simulink model "Mass_Springs_Systems"  (R2021b)
settings: Solver=daessc  StartTime=0.0  StopTime=20  FixedStep=.001  RelTol=1e-3  AbsTol=1e-3  EnableMultiTasking=on
model workspace (MAT data in the model file):
  cslide = 0.25
  iz = [0.192 0.207 0.221 0.238 0.251 0.262 0.268 0.27 0.267 0.262 0.246 0.232 ... (50 elements, 25x2)]
  m1 = 0
  m2 = 0
  m3 = 0
  one = [0.064  0.072; 0.088  0.03; 0.169  0.03; 0.168  0.458; 0.129  0.458; 0.128  0.073]
  smiData : object (value not decoded)
  three = [0.252 0.239 0.214 0.179 0.14 0.107 0.083 0.065 0.075 0.102 0.129 0.163 ... (112 elements, 56x2)]
  two = [0.081 0.042 0.05 0.06 0.082 0.106 0.135 0.161 0.194 0.226 0.253 0.279 ... (72 elements, 36x2)]
  xy_simple = [39.1661  19.7032018238; 3.8339  19.7032; -0.28263658  19.7032; -0.28263658  0; 43  0; 43  19.7032]
  zero = [0.2 0.245 0.288 0.316 0.335 0.345 0.347 0.344 0.338 0.324 0.3 0.269 ... (50 elements, 25x2)]
undefined symbols (not defined in the file): A, d1, d2, ha, sigbuilder_block, X, Y, Z
libraries: sm_lib x7213, nesl_utility x58, simulink x1
(part 2 of 146)

== system Mass_Springs_Systems/Mass Spring Damper Systems ==
  note: 1 Mass 1 Spring
  note: 3 Mass 3 Spring
  note: 2 Mass 2 Spring
  note: 1 Mass 2 Spring
  note: 2 Mass 3 Spring
  note: Equivalent System
  note: Vibrational Machine
  2Masses 2Springs : Subsystem  AncestorBlock=Lib/2Masses 2Springs  VariantControl=22ms  mask{m1=2, m2=1, k1=600, k2=400, d=1, s_f=.35, id1=2, id2=2, zero_forces=on, zerodis=off, force_type=Harmonic, Force=1, Har_Force=1, freq=sqrt(400/1.5)}
      mask prompts: m1 "Mass1 (kg)"; m2 "Mass2 (kg)"; k1 "K1 Spring Constant (N/m)"; k2 "K2 Spring Constant (N/m)"; d "Spring Damping (kg/s)"; s_f "Surface Friction (N/(m/s))"; id1 "M1 Initial Displacement (cm)"; id2 "M2 Initial Displacement (cm)"; zero_forces "Zero Forces"; zerodis "Zero Initial Displacement"; force_type "Force Response Type"; Force "Magnitude(N)"; Har_Force "Magnitude(N)"; freq "Frequency(rad/s)"
      mask init:
      | switch force_type
      |     case 1
      |         Har_Force = 0;
      |         freq = 0;
      |     case 2
      |         Force = 0;
      | end
      | if zero_forces == 1
      |     Har_Force = 0;
      |     Force = 0;
      |     freq = 0;
      | end
      | 
      | if zerodis == 1
      |     id1=0;
      |     id2=0;
      | end
      mask Callback zero_forces:
      | % Enable and disable parameters
      | 
      | % Get the value of the Enable Bias checkbox
      | % unchecked = 'off'
      | % checked = 'on'
      | enab = get_param(gcb,'zero_forces');
      | 
      | % Set the 'MaskEnables' property for each parameters
      | if strcmp(enab,'on')
      |     set_param(gcb,'MaskVisibilities',{'on','on','on','on','on','on','on','on','on','off','off','off','off','off'});
      | else
      |     set_param(gcb,'MaskVisibilities',{'on','on','on','on','on','on','on','on','on','on','on','on','on','on'});
      | end
      | 
      | % Note that the value of the bias is not handled here.
      | % See the Initialization tab
      mask Callback zerodis:
      | % Enable and disable parameters
      | 
      | % Get the value of the Enable Bias checkbox
      | % unchecked = 'off'
      | % checked = 'on'
      | enab = get_param(gcb,'zerodis');
      | 
      | % Set the 'MaskEnables' property for each parameters
      | if strcmp(enab,'on')
      |     set_param(gcb,'MaskEnables',{'on','on','on','on','on','on','off','off','on','on','on','on','on','on'});
      | else
      |     set_param(gcb,'MaskEnables',{'on','on','on','on','on','on','on','on','on','on','on','on','on','on'});
      | end
      | 
      | % Note that the value of the bias is not handled here.
      | % See the Initialization tab
      mask TypeOptions force_type: Step | Harmonic
      mask DialogControl Control4 Prompt: Update Model
      mask DialogControl Control4 Callback: set_param(bdroot,'SimulationCommand','update')
      mask DialogControl Control2 Prompt: Run Simulation
      mask DialogControl Control2 Callback: set_param(bdroot,'SimulationCommand','start')
      mask DialogControl Control3 Prompt: STOP Simulation
      mask DialogControl Control3 Callback: set_param(bdroot,'SimulationCommand','stop')
      mask DialogControl Control7 Prompt: Open Scope Plot
      mask DialogControl Control7 Callback: open(Simulink.BlockPath({'Mass_Springs_Systems/Mass Spring Damper Systems/2Masses 2Springs/Position'}))
      mask DialogControl Control14 Prompt: Frequency Plot
      mask DialogControl Control14 Callback:
      | cart1=evalin('base','out.pos1');
      | cart2=evalin('base','out.pos2');
      | time=evalin('base','out.tout');
      | 
      | Ts = time(2)-time(1);
      | fs = 1/Ts;
      | N = length(cart1);
      | 
      | Y1 = abs(fft(cart1)/N); % fft of cart1 data
      | Y1d = Y1(1:N/2+1); %single side spectrum
      | Y1d(2:end-1) = 2*Y1d(2:end-1); %amplitude adjustment
      | 
      | Y2 = abs(fft(cart2)/N);
      | Y2d = Y2(1:N/2+1);
      | Y2d(2:end-1) = 2*Y2d(2:end-1);
      | 
      | 
      | f = fs*(0:(N/2))/N; %create frequency vector
      | 
      | figure;
      | plot(f,Y1d); xlim([0 10]);
      | hold on;
      | plot(f,Y2d,'r')
      | hold off;
      mask DialogControl Control16 Prompt: Mode Ratios
      mask DialogControl Control16 Callback:
      | syms  w
      | m1=get_param(gcb,'m1');
      | m1=str2double(m1);
      | m2=get_param(gcb,'m2');
      | m2=str2double(m2);
      | k1=get_param(gcb,'k1');
      | k1=str2double(k1);
      | k2=get_param(gcb,'k2');
      | k2=str2double(k2);
      | M=[k1+k2-m1*w^2 -k2; -k2 k2-m2*w^2];
      | detM=det(M);
      | solution=double(solve(detM==0,w));
      | pos=solution>0;
      | wsolution=solution(pos);
      | w1=wsolution(1);
      | w2=wsolution(2);
      | f1=w1/(2*pi);
      | f2=w2/(2*pi);
      | M1=double(subs(M,w,w1));
      | Mode_Ratio_1=M1(1,1)/-M1(1,2);
      | M2=double(subs(M,w,w2));
      | Mode_Ratio_2=M2(1,1)/-M2(1,2);
      | %set_param(gcb,'MaskSelfModifiable','on');
      | % Get the mask object
      | mo = get_param(gcb,'MaskObject');
      | % Get the text object
      | tc = mo.getDialogControl('TextControl1');
      | % Change the string
      | tc.Prompt = string(Mode_Ratio_1);
      | % Get the text object
      | tc = mo.getDialogControl('TextControl2');
      | % Change the string
      | tc.Prompt = string(Mode_Ratio_2);
      mask DialogControl Container6 Prompt: Variables
      mask DialogControl Control13 Prompt: (Add text here)
      mask DialogControl Container8 Prompt: Free Response
      mask DialogControl Container11 Prompt: Free Response
      mask DialogControl Control17 Prompt: Mode Ratio of Mass 1:
      mask DialogControl TextControl1 Prompt: 1.6861
      mask DialogControl Control19 Prompt: Mode Ratio of Mass 2:
      mask DialogControl TextControl2 Prompt: -1.1861
      mask DialogControl Control10 Prompt: "Check Box below for Only Free Response"
      mask DialogControl Container19 Prompt: Forced Response
      mask DialogControl Container10 Prompt: Forced Response
      mask DialogControl Control9 Prompt: Uncheck "Zero Forces" in Free Response Tab to add Forced Response
      mask DialogControl Container13 Prompt: Step Response
      mask DialogControl Container16 Prompt: Harmonic Response
      mask Display: image('$imagefile'); % Use "Edit Image" on toolstrip to change.
  2Masses 3Springs : Subsystem  AncestorBlock=Lib/2Masses 3Springs  VariantControl=23ms  mask{m1=2, m2=2, k1=700, k2=300, k3=700, d=1/3, s_f=0, id1=3.500, id2=-3.500, zero_forces=on, zerodis=off, force_type=Harmonic, Force=5, Har_Force=3, freq=20}
      mask prompts: m1 "Mass1 (kg)"; m2 "Mass2 (kg)"; k1 "K1 Spring Constant (N/m)"; k2 "K2 Spring Constant (N/m)"; k3 "K3 Spring Constant (N/m)"; d "Spring Damping (kg/s)"; s_f "Surface Friction (N/(m/s))"; id1 "M1 Initial Displacement (cm)"; id2 "M2 Initial Displacement (cm)"; zero_forces "Zero Forces"; zerodis "Zero Initial Displacement"; force_type "Force Response Type"; Force "Magnitude(N)"; Har_Force "Magnitude(N)"; freq "Frequency(rad/s)"
      mask init:
      | switch force_type
      |     case 1
      |         Har_Force = 0;
      |         freq = 0;
      |     case 2
      |         Force = 0;
      | end
      | if zero_forces == 1
      |     Har_Force = 0;
      |     Force = 0;
      |     freq = 0;
      | end
      | 
      | if zerodis == 1
      |     id1 = 0;
      |     id2 = 0;
      | end
      mask Callback zero_forces:
      | % Enable and disable parameters
      | 
      | % Get the value of the Enable Bias checkbox
      | % unchecked = 'off'
      | % checked = 'on'
      | enab = get_param(gcb,'zero_forces');
      | 
      | % Set the 'MaskEnables' property for each parameters
      | if strcmp(enab,'on')
      |     set_param(gcb,'MaskVisibilities',{'on','on','on','on','on','on','on','on','on','on','off','off','off','off','off'});
      | else
      |     set_param(gcb,'MaskVisibilities',{'on','on','on','on','on','on','on','on','on','on','on','on','on','on','on'});
      | end
      | 
      | % Note that the value of the bias is not handled here.
      | % See the Initialization tab
      mask Callback zerodis:
      | % Enable and disable parameters
      | 
      | % Get the value of the Enable Bias checkbox
      | % unchecked = 'off'
      | % checked = 'on'
      | enab = get_param(gcb,'zerodis');
      | 
      | % Set the 'MaskEnables' property for each parameters
      | if strcmp(enab,'on')
      |     set_param(gcb,'MaskEnables',{'on','on','on','on','on','on','on','off','off','on','on','on','on','on','on'});
      | else
      |     set_param(gcb,'MaskEnables',{'on','on','on','on','on','on','on','on','on','on','on','on','on','on','on'});
      | end
      | 
      | % Note that the value of the bias is not handled here.
      | % See the Initialization tab
      mask TypeOptions force_type: Step | Harmonic
      mask DialogControl Control4 Prompt: Update Model
      mask DialogControl Control4 Callback: set_param(bdroot,'SimulationCommand','update')
      mask DialogControl Control14 Prompt: Run Simulation
      mask DialogControl Control14 Callback: set_param(bdroot,'SimulationCommand','start')
      mask DialogControl Control3 Prompt: STOP Simulation
      mask DialogControl Control3 Callback: set_param(bdroot,'SimulationCommand','stop')
      mask DialogControl Control7 Prompt: Open Scope Plot
      mask DialogControl Control7 Callback: open(Simulink.BlockPath({'Mass_Springs_Systems/Mass Spring Damper Systems/2Masses 3Springs/Position'}))
      mask DialogControl Control15 Prompt: Frequency Plot
      mask DialogControl Control15 Callback:
      | cart1=evalin('base','out.pos1');
      | cart2=evalin('base','out.pos2');
      | time=evalin('base','out.tout');
      | 
      | Ts = time(2)-time(1);
      | fs = 1/Ts;
      | N = length(cart1);
      | 
      | Y1 = abs(fft(cart1)/N); % fft of cart1 data
      | Y1d = Y1(1:N/2+1); %single side spectrum
      | Y1d(2:end-1) = 2*Y1d(2:end-1); %amplitude adjustment
      | 
      | Y2 = abs(fft(cart2)/N);
      | Y2d = Y2(1:N/2+1);
      | Y2d(2:end-1) = 2*Y2d(2:end-1);
      | 
      | 
      | f = fs*(0:(N/2))/N; %create frequency vector
      | 
      | figure;
      | plot(f,Y1d); xlim([0 10]);
      | hold on;
      | plot(f,Y2d,'r')
      mask DialogControl Control18 Prompt: Mode Ratios
      mask DialogControl Control18 Callback:
      | syms  w
      | m1=get_param(gcb,'m1');
      | m1=str2double(m1);
      | m2=get_param(gcb,'m2');
      | m2=str2double(m2);
      | k1=get_param(gcb,'k1');
      | k1=str2double(k1);
      | k2=get_param(gcb,'k2');
      | k2=str2double(k2);
      | k3=get_param(gcb,'k3');
      | k3=str2double(k3);
      | M=[k1+k2-m1*w^2 -k2; -k2 k2+k3-m2*w^2];
      | detM=det(M);
      | solution=double(solve(detM==0,w));
      | pos=solution>0;
      | wsolution=solution(pos);
      | w1=wsolution(1);
      | w2=wsolution(2);
      | f1=w1/(2*pi);
      | f2=w2/(2*pi);
      | M1=double(subs(M,w,w1)) ;
      | Mode_Ratio_1=M1(1,1)/-M1(1,2);
      | M2=double(subs(M,w,w2)) ;
      | Mode_Ratio_2=M2(1,1)/-M2(1,2);
      | %set_param(gcb,'MaskSelfModifiable','on');
      | % Get the mask object
      | mo = get_param(gcb,'MaskObject');
      | % Get the text object
      | tc = mo.getDialogControl('TextControl1');
      | % Change the string
      | tc.Prompt = string(Mode_Ratio_1);
      | % Get the text object
      | tc = mo.getDialogControl('TextControl2');
      | % Change the string
      | tc.Prompt = string(Mode_Ratio_2);
      mask DialogControl Container6 Prompt: Variables
      mask DialogControl Container8 Prompt: Free Response
      mask DialogControl Container11 Prompt: Free Response
      mask DialogControl Control21 Prompt: Mode Ratio of Mass1:
      mask DialogControl TextControl1 Prompt: 1
      mask DialogControl Control22 Prompt: Mode Ratio of Mass 2:
      mask DialogControl TextControl2 Prompt: -1
      mask DialogControl Control10 Prompt: "Check Box below for Only Free Response"
      mask DialogControl Container19 Prompt: Forced Response
      mask DialogControl Container10 Prompt: Forced Response
      mask DialogControl Control9 Prompt: Uncheck "Zero Forces" in Free Response Tab to add Forced Response
      mask DialogControl Container13 Prompt: Step Response
      mask DialogControl Container16 Prompt: Harmonic Response
      mask Display: image('$imagefile'); % Use "Edit Image" on toolstrip to change.
  3Masses 3Springs : Subsystem  AncestorBlock=Lib/3Masses 3Springs  VariantControl=33ms  mask{m1=1, m2=1, m3=1, k1=100, k2=100, k3=100, d=1, s_f=0, d1=3.500, d2=3.500, d3=3.500, zero_forces=off, zerodis=off, force_type=Step, Force=5, Har_Force=6, freq=20}
      mask prompts: m1 "Mass1 (kg)"; m2 "Mass2 (kg)"; m3 "Mass3 (kg)"; k1 "K1 Spring Constant (N/m)"; k2 "K2 Spring Constant (N/m)"; k3 "K3 Spring Constant (N/m)"; d "Spring Damping (kg/s)"; s_f "Surface Friction (N/(m/s))"; d1 "M1 Initial Displacement (cm)"; d2 "M2 Initial Displacement (cm)"; d3 "M3 Initial Displacement (cm)"; zero_forces "Zero Forces"; zerodis "Zero Initial Displacement"; force_type "Force Response Type"; Force "Magnitude(N)"; Har_Force "Magnitude(N)"; freq "Frequency(rad/s)"
      mask init:
      | switch force_type
      |     case 1
      |         Har_Force = 0;
      |         freq = 0;
      |     case 2
      |         Force = 0;
      | end
      | if zero_forces == 1
      |     Har_Force = 0;
      |     Force = 0;
      |     freq = 0;
      | end
      | 
      | if zerodis == 1
      |     id1 = 0;
      |     id2 = 0;
      |     id3 = 0;
      | end
      mask Callback zero_forces:
      | % Enable and disable parameters
      | 
      | % Get the value of the Enable Bias checkbox
      | % unchecked = 'off'
      | % checked = 'on'
      | enab = get_param(gcb,'zero_forces');
      | 
      | % Set the 'MaskEnables' property for each parameters
      | if strcmp(enab,'on')
      |     set_param(gcb,'MaskVisibilities',{'on','on','on','on','on','on','on','on','on','on','on','on','off','off','off','off','off'});
      | else
      |     set_param(gcb,'MaskVisibilities',{'on','on','on','on','on','on','on','on','on','on','on','on','on','on','on','on','on'});
      | end
      | 
      | % Note that the value of the bias is not handled here.
      | % See the Initialization tab
      mask Callback zerodis:
      | % Enable and disable parameters
      | 
      | % Get the value of the Enable Bias checkbox
      | % unchecked = 'off'
      | % checked = 'on'
      | enab = get_param(gcb,'zerodis');
      | 
      | % Set the 'MaskEnables' property for each parameters
      | if strcmp(enab,'on')
      |     set_param(gcb,'MaskEnables',{'on','on','on','on','on','on','on','on','off','off','off','on','on','on','on','on','on'});
      | else
      |     set_param(gcb,'MaskEnables',{'on','on','on','on','on','on','on','on','on','on','on','on','on','on','on','on','on'});
      | end
      | 
      | % Note that the value of the bias is not handled here.
      | % See the Initialization tab
      mask TypeOptions force_type: Step | Harmonic
      mask DialogControl Control4 Prompt: Update Model
      mask DialogControl Control4 Callback: set_param(bdroot,'SimulationCommand','update')
      mask DialogControl Control2 Prompt: Run Simulation
      mask DialogControl Control2 Callback: set_param(bdroot,'SimulationCommand','start')
      mask DialogControl Control3 Prompt: STOP Simulation
      mask DialogControl Control3 Callback: set_param(bdroot,'SimulationCommand','stop')
      mask DialogControl Control7 Prompt: Open Scope Plot
      mask DialogControl Control7 Callback: open(Simulink.BlockPath({'Mass_Springs_Systems/Mass Spring Damper Systems/3Masses 3Springs/Position'}))
      mask DialogControl Control14 Prompt: Frequency Plot
      mask DialogControl Control14 Callback:
      | cart1=evalin('base','out.pos1');
      | cart2=evalin('base','out.pos2');
      | cart3=evalin('base','out.pos3');
      | time=evalin('base','out.tout');
      | 
      | Ts = time(2)-time(1);
      | fs = 1/Ts;
      | N = length(cart1);
      | 
      | Y1 = abs(fft(cart1)/N); % fft of cart1 data
      | Y1d = Y1(1:N/2+1); %single side spectrum
      | Y1d(2:end-1) = 2*Y1d(2:end-1); %amplitude adjustment
      | 
      | Y2 = abs(fft(cart2)/N);
      | Y2d = Y2(1:N/2+1);
      | Y2d(2:end-1) = 2*Y2d(2:end-1);
      | 
      | Y3 = abs(fft(cart3)/N);
      | Y3d = Y3(1:N/2+1);
      | Y3d(2:end-1) = 2*Y3d(2:end-1);
      | 
      | f = fs*(0:(N/2))/N; %create frequency vector
      | 
      | figure;
      | plot(f,Y1d); xlim([0 10]);
      | hold on;
      | plot(f,Y2d,'r')
      | plot(f,Y3d,'g')
      mask DialogControl Container6 Prompt: Variables
      mask DialogControl Container8 Prompt: Free Response
      mask DialogControl Container11 Prompt: Free Response
      mask DialogControl Control10 Prompt: "Check Box below for Only Free Response"
      mask DialogControl Container19 Prompt: Forced Response
      mask DialogControl Container10 Prompt: Forced Response
      mask DialogControl Control9 Prompt: Uncheck "Zero Forces" in Free Response Tab to add Forced Response
      mask DialogControl Container13 Prompt: Step Response
      mask DialogControl Container16 Prompt: Harmonic Response
      mask Display: image('$imagefile'); % Use "Edit Image" on toolstrip to change.
  Equivalent System : Subsystem  VariantControl=ES  mask{length=20, b_thk=2.8, tip_mass=0, materials=TPU, den=.88, ymod=3.5, pr=.3, t_spr1=off, top_spr1_stiff=10, top_spr1_dpg=0, t_spr2=off, top_spr2_stiff=50, top_spr2_dpg=.00001, t_spr3=off, top_spr3_stiff=20, top_spr3_dpg=0, t_spr4=on, top_spr4_stiff=50, top_spr4_dpg=.00001, b_spr1=off, bottom_spr1_stiff=10, bottom_spr1_dpg=1, b_spr2=off, bottom_spr2_stiff=0, bottom_spr2_dpg=0, b_spr3=off, bottom_spr3_stiff=.5, bottom_spr3_dpg=0.00001, b_spr4=off, bottom_spr4_stiff=.5, bottom_spr4_dpg=0, theta=-4.800, zerodis=off, freeforce=on, type_force=Harmonic, Force=2, Har_Force=2, freq=5, Imp_Force=1, meq=1, keq=100, ceq=1}
      mask prompts: length "Beam Length (cm)"; b_thk "Beam Thickness (mm)"; tip_mass "Load Mass (g)"; materials "Beam Material"; den "Density (g/cm^3)"; ymod "Young's Modulus (GPa)"; pr "Poisson's Ratio"; t_spr1 "Spring 1"; top_spr1_stiff "Stiffness (N/m)"; top_spr1_dpg "Damping (N/m)"; t_spr2 "Spring 2"; top_spr2_stiff "Stiffness (N/m)"; top_spr2_dpg "Damping (N/m)"; t_spr3 "Spring 3"; top_spr3_stiff "Stiffness (N/m)"; top_spr3_dpg "Damping (N/m)"; t_spr4 "Spring 4"; top_spr4_stiff "Stiffness (N/m)"; top_spr4_dpg "Damping (N/m)"; b_spr1 "Spring 1"; bottom_spr1_stiff "Stiffness (N/m)"; bottom_spr1_dpg "Damping (N/m)"; b_spr2 "Spring 2"; bottom_spr2_stiff "Stiffness (N/m)"; bottom_spr2_dpg "Damping (N/m)"; b_spr3 "Spring 3"; bottom_spr3_stiff "Stiffness (N/m)"; bottom_spr3_dpg "Damping (N/m)"; b_spr4 "Spring 4"; bottom_spr4_stiff "Stiffness (N/m)"; bottom_spr4_dpg "Damping (N/m)"; theta "Inital Displacement of Beam (deg):"; zerodis "Zero Initial Displacement"; freeforce "Zero Forces"; type_force "Force Response Type"; Force "Magnitude (N):"; Har_Force "Magnitude (N):"; freq "Frequency (rad/s):"; Imp_Force "Magnitude (N):"; meq "Equivalent Mass (kg):"; keq "Equivalent Stiffness (N/m):"; ceq "Equivalent Damping (N/m):"
      mask init:
      | t1ih=(1/4)*length*tand(-theta)*.01;
      | t2ih=(2/4)*length*tand(-theta)*.01;
      | t3ih=(3/4)*length*tand(-theta)*.01;
      | t4ih=length*tand(-theta)*.01;
      | b1ih=(1/4)*length*tand(theta)*.01;
      | b2ih=(2/4)*length*tand(theta)*.01;
      | b3ih=(3/4)*length*tand(theta)*.01;
      | b4ih=length*tand(theta)*.01;
      | 
      | thetaeq = -length*tand(theta)*.01;
      | switch materials
      |     case 1
      |         b_stff = 259;
      |         b_damping = .013;
      |         b_density= 7.85;
      | %        b_ymod= 200e9;
      | %         b_pr= .285;
      |     case 2
      |         b_stff = 3.27;
      |         b_damping = .00056;
      |         b_density= 1.2;
      | %        b_ymod= 2.53e9;
      | %         b_pr= .33;
      |     case 3
      |         b_stff = 4.522;
      |         b_damping = .000675;
      |         b_density= 1.24;
      | %        b_ymod= 3.5e9;
      | %         b_pr= .3;
      |     case 4
      |         b_stff = 2.59725;
      |         b_damping = .000515;
      |         b_density= 1.23;
      | %        b_ymod= 2.01e9;
      | %         b_pr= .32;
      |     case 5
      |         Ia = (.025*(b_thk*10^-3)^3)/12;
      |         l = length*10^-2/4;
      |         b_stff = (ymod*10^9*Ia)/l;
      |         b_damping = .0001*2*b_stff;
      |         b_density = den;
      | end
      | switch type_force
      |     case 1,
      |         Imp_Force=0;
      |         Har_Force=0;
      |         freq=0;
      |     case 2,
      |         Force=0;
      |         Imp_Force=0;
      |     case 3
      |         Force=0;
      |         Har_Force=0;
      |         freq=0;
      |     otherwise, assert(false);
      | end
      | if freeforce == 1
      |     Force = 0;
      |     Har_Force = 0;
      |     Imp_Force = 0;
      | end
      | 
      | if zerodis == 1
      |     t1ih= 0;
      |     t2ih= 0;
      |     t3ih= 0;
      |     t4ih= 0;
      |     b1ih= 0;
      |     b2ih= 0;
      |     b3ih= 0;
      |     b4ih= 0;
      |     theta=0;
      | end
      mask TypeOptions materials: Steel | TPU | PLA | PETG | Enter Material Properties
      mask Callback materials:
      | %Getting cell of blocks
      | parnum1 = find(strcmp(get_param('Mass_Springs_Systems/Mass Spring Damper Systems/Equivalent System','MaskNames'),'den'));
      | parnum2 = find(strcmp(get_param('Mass_Springs_Systems/Mass Spring Damper Systems/Equivalent System','MaskNames'),'ymod'));
      | parnum3 = find(strcmp(get_param('Mass_Springs_Systems/Mass Spring Damper Systems/Equivalent System','MaskNames'),'dpr'));
      | 
      | % Checking if Checkbox is marked duh
      | x = get_param(gcb,'materials');
      | 
      | if strcmp(x,'Enter Material Properties')
      |     me1 = get_param('Mass_Springs_Systems/Mass Spring Damper Systems/Equivalent System', 'MaskVisibilities');
      |     me1{5} = 'on';
      |     me1{6} = 'on';
      |     me1{7} = 'on';
      |     set_param('Mass_Springs_Systems/Mass Spring Damper Systems/Equivalent System', 'MaskVisibilities',me1);
      | 
      | else
      |     me1 = get_param('Mass_Springs_Systems/Mass Spring Damper Systems/Equivalent System', 'MaskVisibilities');
      |     me1{5} = 'off';
      |     me1{6} = 'off';
      |     me1{7} = 'off';
      |     set_param('Mass_Springs_Systems/Mass Spring Damper Systems/Equivalent System', 'MaskVisibilities',me1);
      | 
      | end
      mask Callback t_spr1:
      | commswtspr1 = get_param(gcb,'t_spr1');
      | x = get_param(gcb,'t_spr1');
      | if strcmp(x,'on')
      |     me1 = get_param('Mass_Springs_Systems/Mass Spring Damper Systems/Equivalent System', 'MaskVisibilities');
      |     me1{9} = 'on';
      |     me1{10} = 'on';
      |     set_param('Mass_Springs_Systems/Mass Spring Damper Systems/Equivalent System', 'MaskVisibilities',me1);
      | else
      |     me1 = get_param('Mass_Springs_Systems/Mass Spring Damper Systems/Equivalent System', 'MaskVisibilities');
      |     me1{9} = 'off';
      |     me1{10} = 'off';
      |     set_param('Mass_Springs_Systems/Mass Spring Damper Systems/Equivalent System', 'MaskVisibilities',me1);
      | end
      | if strcmp(commswtspr1,'on')
      |     set_param('Mass_Springs_Systems/Mass Spring Damper Systems/Equivalent System/RT tspr1','Commented','off');
      |     set_param('Mass_Springs_Systems/Mass Spring Damper Systems/Equivalent System/TRT1Rev1','Commented','off');
      |     set_param('Mass_Springs_Systems/Mass Spring Damper Systems/Equivalent System/TRev1','Commented','off');
      |     set_param('Mass_Springs_Systems/Mass Spring Damper Systems/Equivalent System/TRT1Rev2','Commented','off');
      |     set_param('Mass_Springs_Systems/Mass Spring Damper Systems/Equivalent System/tspr1','Commented','off');
      |     set_param('Mass_Springs_Systems/Mass Spring Damper Systems/Equivalent System/SJ tspr1','Commented','off');
      | else
      |     set_param('Mass_Springs_Systems/Mass Spring Damper Systems/Equivalent System/RT tspr1','Commented','on');
      |     set_param('Mass_Springs_Systems/Mass Spring Damper Systems/Equivalent System/TRT1Rev1','Commented','on');
      |     set_param('Mass_Springs_Systems/Mass Spring Damper Systems/Equivalent System/TRev1','Commented','on');
      |     set_param('Mass_Springs_Systems/Mass Spring Damper Systems/Equivalent System/TRT1Rev2','Commented','on');
      |     set_param('Mass_Springs_Systems/Mass Spring Damper Systems/Equivalent System/tspr1','Commented','on');
      |     set_param('Mass_Springs_Systems/Mass Spring Damper Systems/Equivalent System/SJ tspr1','Commented','on');
      | end
      mask Callback t_spr2:
      | commswtspr2 = get_param(gcb,'t_spr2');
      | x = get_param(gcb,'t_spr2');
      | if strcmp(x,'on')
      |     me1 = get_param('Mass_Springs_Systems/Mass Spring Damper Systems/Equivalent System', 'MaskVisibilities');
      |     me1{12} = 'on';
      |     me1{13} = 'on';
      |     set_param('Mass_Springs_Systems/Mass Spring Damper Systems/Equivalent System', 'MaskVisibilities',me1);
      | else
      |     me1 = get_param('Mass_Springs_Systems/Mass Spring Damper Systems/Equivalent System', 'MaskVisibilities');
      |     me1{12} = 'off';
      |     me1{13} = 'off';
      |     set_param('Mass_Springs_Systems/Mass Spring Damper Systems/Equivalent System', 'MaskVisibilities',me1);
      | end
      | if strcmp(commswtspr2,'on')
      |     set_param('Mass_Springs_Systems/Mass Spring Damper Systems/Equivalent System/RT tspr2','Commented','off');
      |     set_param('Mass_Springs_Systems/Mass Spring Damper Systems/Equivalent System/TRT2Rev1','Commented','off');
      |     set_param('Mass_Springs_Systems/Mass Spring Damper Systems/Equivalent System/TRev2','Commented','off');
      |     set_param('Mass_Springs_Systems/Mass Spring Damper Systems/Equivalent System/TRT2Rev2','Commented','off');
      |     set_param('Mass_Springs_Systems/Mass Spring Damper Systems/Equivalent System/tspr2','Commented','off');
      |     set_param('Mass_Springs_Systems/Mass Spring Damper Systems/Equivalent System/SJ tspr2','Commented','off');
      | else
      |     set_param('Mass_Springs_Systems/Mass Spring Damper Systems/Equivalent System/RT tspr2','Commented','on');
      |     set_param('Mass_Springs_Systems/Mass Spring Damper Systems/Equivalent System/TRT2Rev1','Commented','on');
      |     set_param('Mass_Springs_Systems/Mass Spring Damper Systems/Equivalent System/TRev2','Commented','on');
      |     set_param('Mass_Springs_Systems/Mass Spring Damper Systems/Equivalent System/TRT2Rev2','Commented','on');
      |     set_param('Mass_Springs_Systems/Mass Spring Damper Systems/Equivalent System/tspr2','Commented','on');
      |     set_param('Mass_Springs_Systems/Mass Spring Damper Systems/Equivalent System/SJ tspr2','Commented','on');
      | end
      mask Callback t_spr3:
      | commswtspr3 = get_param(gcb,'t_spr3');
      | x = get_param(gcb,'t_spr3');
      | if strcmp(x,'on')
      |     me1 = get_param('Mass_Springs_Systems/Mass Spring Damper Systems/Equivalent System', 'MaskVisibilities');
      |     me1{15} = 'on';
      |     me1{16} = 'on';
      |     set_param('Mass_Springs_Systems/Mass Spring Damper Systems/Equivalent System', 'MaskVisibilities',me1);
      | else
      |     me1 = get_param('Mass_Springs_Systems/Mass Spring Damper Systems/Equivalent System', 'MaskVisibilities');
      |     me1{15} = 'off';
      |     me1{16} = 'off';
      |     set_param('Mass_Springs_Systems/Mass Spring Damper Systems/Equivalent System', 'MaskVisibilities',me1);
      | end
      | if strcmp(commswtspr3,'on')
      |     set_param('Mass_Springs_Systems/Mass Spring Damper Systems/Equivalent System/RT tspr3','Commented','off');
      |     set_param('Mass_Springs_Systems/Mass Spring Damper Systems/Equivalent System/TRT3Rev1','Commented','off');
      |     set_param('Mass_Springs_Systems/Mass Spring Damper Systems/Equivalent System/TRev3','Commented','off');
      |     set_param('Mass_Springs_Systems/Mass Spring Damper Systems/Equivalent System/TRT3Rev2','Commented','off');
      |     set_param('Mass_Springs_Systems/Mass Spring Damper Systems/Equivalent System/tspr3','Commented','off');
      |     set_param('Mass_Springs_Systems/Mass Spring Damper Systems/Equivalent System/SJ tspr3','Commented','off');
      | else
      |     set_param('Mass_Springs_Systems/Mass Spring Damper Systems/Equivalent System/RT tspr3','Commented','on');
      |     set_param('Mass_Springs_Systems/Mass Spring Damper Systems/Equivalent System/TRT3Rev1','Commented','on');
      |     set_param('Mass_Springs_Systems/Mass Spring Damper Systems/Equivalent System/TRev3','Commented','on');
      |     set_param('Mass_Springs_Systems/Mass Spring Damper Systems/Equivalent System/TRT3Rev2','Commented','on');
      |     set_param('Mass_Springs_Systems/Mass Spring Damper Systems/Equivalent System/tspr3','Commented','on');
      |     set_param('Mass_Springs_Systems/Mass Spring Damper Systems/Equivalent System/SJ tspr3','Commented','on');
      | end
      mask Callback t_spr4:
      | commswtspr4 = get_param(gcb,'t_spr4');
      | x = get_param(gcb,'t_spr4');
      | if strcmp(x,'on')
      |     me1 = get_param('Mass_Springs_Systems/Mass Spring Damper Systems/Equivalent System', 'MaskVisibilities');
      |     me1{18} = 'on';
      |     me1{19} = 'on';
      |     set_param('Mass_Springs_Systems/Mass Spring Damper Systems/Equivalent System', 'MaskVisibilities',me1);
      | else
      |     me1 = get_param('Mass_Springs_Systems/Mass Spring Damper Systems/Equivalent System', 'MaskVisibilities');
      |     me1{18} = 'off';
      |     me1{19} = 'off';
      |     set_param('Mass_Springs_Systems/Mass Spring Damper Systems/Equivalent System', 'MaskVisibilities',me1);
      | end
      | if strcmp(commswtspr4,'on')
      |     set_param('Mass_Springs_Systems/Mass Spring Damper Systems/Equivalent System/RT tspr4','Commented','off');
      |     set_param('Mass_Springs_Systems/Mass Spring Damper Systems/Equivalent System/TRT4Rev1','Commented','off');
      |     set_param('Mass_Springs_Systems/Mass Spring Damper Systems/Equivalent System/TRev4','Commented','off');
      |     set_param('Mass_Springs_Systems/Mass Spring Damper Systems/Equivalent System/TRT4Rev2','Commented','off');
      |     set_param('Mass_Springs_Systems/Mass Spring Damper Systems/Equivalent System/tspr4','Commented','off');
      |     set_param('Mass_Springs_Systems/Mass Spring Damper Systems/Equivalent System/SJ tspr4','Commented','off');
      | else
      |     set_param('Mass_Springs_Systems/Mass Spring Damper Systems/Equivalent System/RT tspr4','Commented','on');
      |     set_param('Mass_Springs_Systems/Mass Spring Damper Systems/Equivalent System/TRT4Rev1','Commented','on');
      |     set_param('Mass_Springs_Systems/Mass Spring Damper Systems/Equivalent System/TRev4','Commented','on');
      |     set_param('Mass_Springs_Systems/Mass Spring Damper Systems/Equivalent System/TRT4Rev2','Commented','on');
      |     set_param('Mass_Springs_Systems/Mass Spring Damper Systems/Equivalent System/tspr4','Commented','on');
      |     set_param('Mass_Springs_Systems/Mass Spring Damper Systems/Equivalent System/SJ tspr4','Commented','on');
      | end
      mask Callback b_spr1:
      | commswbspr1 = get_param(gcb,'b_spr1');
      | x = get_param(gcb,'b_spr1');
      | if strcmp(x,'on')
      |     me1 = get_param('Mass_Springs_Systems/Mass Spring Damper Systems/Equivalent System', 'MaskVisibilities');
      |     me1{21} = 'on';
      |     me1{22} = 'on';
      |     set_param('Mass_Springs_Systems/Mass Spring Damper Systems/Equivalent System', 'MaskVisibilities',me1);
      | else
      |     me1 = get_param('Mass_Springs_Systems/Mass Spring Damper Systems/Equivalent System', 'MaskVisibilities');
      |     me1{21} = 'off';
      |     me1{22} = 'off';
      |     set_param('Mass_Springs_Systems/Mass Spring Damper Systems/Equivalent System', 'MaskVisibilities',me1);
      | end
      | if strcmp(commswbspr1,'on')
      |     set_param('Mass_Springs_Systems/Mass Spring Damper Systems/Equivalent System/RT bspr1','Commented','off');
      |     set_param('Mass_Springs_Systems/Mass Spring Damper Systems/Equivalent System/BRT1Rev1','Commented','off');
      |     set_param('Mass_Springs_Systems/Mass Spring Damper Systems/Equivalent System/BRev1','Commented','off');
      |     set_param('Mass_Springs_Systems/Mass Spring Damper Systems/Equivalent System/BRT1Rev2','Commented','off');
      |     set_param('Mass_Springs_Systems/Mass Spring Damper Systems/Equivalent System/bspr1','Commented','off');
      |     set_param('Mass_Springs_Systems/Mass Spring Damper Systems/Equivalent System/SJ bspr1','Commented','off');
      | else
      |     set_param('Mass_Springs_Systems/Mass Spring Damper Systems/Equivalent System/RT bspr1','Commented','on');
      |     set_param('Mass_Springs_Systems/Mass Spring Damper Systems/Equivalent System/BRT1Rev1','Commented','on');
      |     set_param('Mass_Springs_Systems/Mass Spring Damper Systems/Equivalent System/BRev1','Commented','on');
      |     set_param('Mass_Springs_Systems/Mass Spring Damper Systems/Equivalent System/BRT1Rev2','Commented','on');
      |     set_param('Mass_Springs_Systems/Mass Spring Damper Systems/Equivalent System/bspr1','Commented','on');
      |     set_param('Mass_Springs_Systems/Mass Spring Damper Systems/Equivalent System/SJ bspr1','Commented','on');
      | end
      mask Callback b_spr2:
      | commswbspr2 = get_param(gcb,'b_spr2');
      | x = get_param(gcb,'b_spr2');
      | if strcmp(x,'on')
      |     me1 = get_param('Mass_Springs_Systems/Mass Spring Damper Systems/Equivalent System', 'MaskVisibilities');
      |     me1{24} = 'on';
      |     me1{25} = 'on';
      |     set_param('Mass_Springs_Systems/Mass Spring Damper Systems/Equivalent System', 'MaskVisibilities',me1);
      | else
      |     me1 = get_param('Mass_Springs_Systems/Mass Spring Damper Systems/Equivalent System', 'MaskVisibilities');
      |     me1{24} = 'off';
      |     me1{25} = 'off';
      |     set_param('Mass_Springs_Systems/Mass Spring Damper Systems/Equivalent System', 'MaskVisibilities',me1);
      | end
      | if strcmp(commswbspr2,'on')
      |     set_param('Mass_Springs_Systems/Mass Spring Damper Systems/Equivalent System/RT bspr2','Commented','off');
      |     set_param('Mass_Springs_Systems/Mass Spring Damper Systems/Equivalent System/BRT2Rev1','Commented','off');
      |     set_param('Mass_Springs_Systems/Mass Spring Damper Systems/Equivalent System/BRev2','Commented','off');
      |     set_param('Mass_Springs_Systems/Mass Spring Damper Systems/Equivalent System/BRT2Rev2','Commented','off');
      |     set_param('Mass_Springs_Systems/Mass Spring Damper Systems/Equivalent System/bspr2','Commented','off');
      |     set_param('Mass_Springs_Systems/Mass Spring Damper Systems/Equivalent System/SJ bspr2','Commented','off');
      | else
      |     set_param('Mass_Springs_Systems/Mass Spring Damper Systems/Equivalent System/RT bspr2','Commented','on');
      |     set_param('Mass_Springs_Systems/Mass Spring Damper Systems/Equivalent System/BRT2Rev1','Commented','on');
      |     set_param('Mass_Springs_Systems/Mass Spring Damper Systems/Equivalent System/BRev2','Commented','on');
      |     set_param('Mass_Springs_Systems/Mass Spring Damper Systems/Equivalent System/BRT2Rev2','Commented','on');
      |     set_param('Mass_Springs_Systems/Mass Spring Damper Systems/Equivalent System/bspr2','Commented','on');
      |     set_param('Mass_Springs_Systems/Mass Spring Damper Systems/Equivalent System/SJ bspr2','Commented','on');
      | end
      mask Callback b_spr3:
      | commswbspr3 = get_param(gcb,'b_spr3');
      | x = get_param(gcb,'b_spr3');
      | if strcmp(x,'on')
      |     me1 = get_param('Mass_Springs_Systems/Mass Spring Damper Systems/Equivalent System', 'MaskVisibilities');
      |     me1{27} = 'on';
      |     me1{28} = 'on';
      |     set_param('Mass_Springs_Systems/Mass Spring Damper Systems/Equivalent System', 'MaskVisibilities',me1);
      | else
      |     me1 = get_param('Mass_Springs_Systems/Mass Spring Damper Systems/Equivalent System', 'MaskVisibilities');
      |     me1{27} = 'off';
      |     me1{28} = 'off';
      |     set_param('Mass_Springs_Systems/Mass Spring Damper Systems/Equivalent System', 'MaskVisibilities',me1);
      | end
      | if strcmp(commswbspr3,'on')
      |     set_param('Mass_Springs_Systems/Mass Spring Damper Systems/Equivalent System/RT bspr3','Commented','off');
      |     set_param('Mass_Springs_Systems/Mass Spring Damper Systems/Equivalent System/BRT3Rev1','Commented','off');
      |     set_param('Mass_Springs_Systems/Mass Spring Damper Systems/Equivalent System/BRev3','Commented','off');
      |     set_param('Mass_Springs_Systems/Mass Spring Damper Systems/Equivalent System/BRT3Rev2','Commented','off');
      |     set_param('Mass_Springs_Systems/Mass Spring Damper Systems/Equivalent System/bspr3','Commented','off');
      |     set_param('Mass_Springs_Systems/Mass Spring Damper Systems/Equivalent System/SJ bspr3','Commented','off');
      | else
      |     set_param('Mass_Springs_Systems/Mass Spring Damper Systems/Equivalent System/RT bspr3','Commented','on');
      |     set_param('Mass_Springs_Systems/Mass Spring Damper Systems/Equivalent System/BRT3Rev1','Commented','on');
      |     set_param('Mass_Springs_Systems/Mass Spring Damper Systems/Equivalent System/BRev3','Commented','on');
      |     set_param('Mass_Springs_Systems/Mass Spring Damper Systems/Equivalent System/BRT3Rev2','Commented','on');
      |     set_param('Mass_Springs_Systems/Mass Spring Damper Systems/Equivalent System/bspr3','Commented','on');
      |     set_param('Mass_Springs_Systems/Mass Spring Damper Systems/Equivalent System/SJ bspr3','Commented','on');
      | end
      mask Callback b_spr4:
      | commswbspr4 = get_param(gcb,'b_spr4');
      | x = get_param(gcb,'b_spr4');
      | if strcmp(x,'on')
      |     me1 = get_param('Mass_Springs_Systems/Mass Spring Damper Systems/Equivalent System', 'MaskVisibilities');
      |     me1{30} = 'on';
      |     me1{31} = 'on';
      |     set_param('Mass_Springs_Systems/Mass Spring Damper Systems/Equivalent System', 'MaskVisibilities',me1);
      | else
      |     me1 = get_param('Mass_Springs_Systems/Mass Spring Damper Systems/Equivalent System', 'MaskVisibilities');
      |     me1{30} = 'off';
      |     me1{31} = 'off';
      |     set_param('Mass_Springs_Systems/Mass Spring Damper Systems/Equivalent System', 'MaskVisibilities',me1);
      | end
      | if strcmp(commswbspr4,'on')
      |     set_param('Mass_Springs_Systems/Mass Spring Damper Systems/Equivalent System/RT bspr4','Commented','off');
      |     set_param('Mass_Springs_Systems/Mass Spring Damper Systems/Equivalent System/BRT4Rev1','Commented','off');
      |     set_param('Mass_Springs_Systems/Mass Spring Damper Systems/Equivalent System/BRev4','Commented','off');
      |     set_param('Mass_Springs_Systems/Mass Spring Damper Systems/Equivalent System/BRT4Rev2','Commented','off');
      |     set_param('Mass_Springs_Systems/Mass Spring Damper Systems/Equivalent System/bspr4','Commented','off');
      |     set_param('Mass_Springs_Systems/Mass Spring Damper Systems/Equivalent System/SJ bspr4','Commented','off');
      | else
      |     set_param('Mass_Springs_Systems/Mass Spring Damper Systems/Equivalent System/RT bspr4','Commented','on');
      |     set_param('Mass_Springs_Systems/Mass Spring Damper Systems/Equivalent System/BRT4Rev1','Commented','on');
      |     set_param('Mass_Springs_Systems/Mass Spring Damper Systems/Equivalent System/BRev4','Commented','on');
      |     set_param('Mass_Springs_Systems/Mass Spring Damper Systems/Equivalent System/BRT4Rev2','Commented','on');
      |     set_param('Mass_Springs_Systems/Mass Spring Damper Systems/Equivalent System/bspr4','Commented','on');
      |     set_param('Mass_Springs_Systems/Mass Spring Damper Systems/Equivalent System/SJ bspr4','Commented','on');
      | end
      mask Callback zerodis:
      | x = get_param(gcb,'zerodis');
      | if strcmp(x,'on')
      |     me1 = get_param('Mass_Springs_Systems/Mass Spring Damper Systems/Equivalent System', 'MaskEnables');
      |     me1{32} = 'off';
      |     set_param('Mass_Springs_Systems/Mass Spring Damper Systems/Equivalent System', 'MaskEnables',me1);
      | else
      |     me1 = get_param('Mass_Springs_Systems/Mass Spring Damper Systems/Equivalent System', 'MaskEnables');
      |     me1{32} = 'on';
      |     set_param('Mass_Springs_Systems/Mass Spring Damper Systems/Equivalent System', 'MaskEnables',me1);
      | end
      mask Callback freeforce:
      | x = get_param(gcb,'freeforce');
      | if strcmp(x,'on')
      |     me1 = get_param('Mass_Springs_Systems/Mass Spring Damper Systems/Equivalent System', 'MaskEnables');
      |     me1{35} = 'off';
      |     me1{36} = 'off';
      |     me1{37} = 'off';
      |     me1{38} = 'off';
      |     me1{39} = 'off';
      |     set_param('Mass_Springs_Systems/Mass Spring Damper Systems/Equivalent System', 'MaskEnables',me1);
      | else
      |     me1 = get_param('Mass_Springs_Systems/Mass Spring Damper Systems/Equivalent System', 'MaskEnables');
      |     me1{35} = 'on';
      |     me1{36} = 'on';
      |     me1{37} = 'on';
      |     me1{38} = 'on';
      |     me1{39} = 'on';
      |     set_param('Mass_Springs_Systems/Mass Spring Damper Systems/Equivalent System', 'MaskEnables',me1);
      | end
      mask TypeOptions type_force: Step | Harmonic | Impulse
      mask DialogControl Control2 Prompt: Update Model
      mask DialogControl Control2 Callback: set_param(bdroot,'SimulationCommand','update')
      mask DialogControl Control3 Prompt: Run Simulation
      mask DialogControl Control3 Callback: set_param(bdroot,'SimulationCommand','start')
      mask DialogControl Control4 Prompt: STOP Simulation
      mask DialogControl Control4 Callback: set_param(bdroot,'SimulationCommand','stop')
      mask DialogControl Control5 Prompt: Open Deflection Plot
      mask DialogControl Control5 Callback: open(Simulink.BlockPath({'Mass_Springs_Systems/Mass Spring Damper Systems/Equivalent System/Deflection'}))
      mask DialogControl Control13 Prompt: Open Angular Deflection Plot
      mask DialogControl Control13 Callback: open(Simulink.BlockPath({'Mass_Springs_Systems/Mass Spring Damper Systems/Equivalent System/Angular Deflection'}))
      mask DialogControl Container4 Prompt: Beam Properties
      mask DialogControl Container27 Prompt: Beam Material
      mask DialogControl Container11 Prompt: Spring Configuration
      mask DialogControl Control10 Prompt: Check the boxes for the springs you want in the model.
      mask DialogControl Container12 Prompt: Top Springs
      mask DialogControl Container32 Prompt: Spring 1
      mask DialogControl Container33 Prompt: Spring 2
      mask DialogControl Container34 Prompt: Spring 3
      mask DialogControl Container35 Prompt: Spring 4
      mask DialogControl Container13 Prompt: Bottom Srings
      mask DialogControl Container36 Prompt: Spring 1
      mask DialogControl Container37 Prompt: Spring 2
      mask DialogControl Container38 Prompt: Spring 3
      mask DialogControl Container39 Prompt: Spring 4
      mask DialogControl Container31 Prompt: Free Response
      mask DialogControl Control12 Prompt: Uncheck "Zero Forces" in Free Response Tab to add Forced Response
      mask DialogControl Container10 Prompt: Force Response
      mask DialogControl Control8 Prompt: "Check Box below for Only Free Response"
      mask DialogControl Container28 Prompt: Step Response
      mask DialogControl Container29 Prompt: Harmonic Response
      mask DialogControl Container30 Prompt: Impulse Response
      mask DialogControl Container25 Prompt: Equivalent System
      mask DialogControl Control15 Prompt: Open Comparison Plot
      mask DialogControl Control15 Callback: open(Simulink.BlockPath({'Mass_Springs_Systems/Mass Spring Damper Systems/Equivalent System/Comparison Plot'}))
      mask Display: image('$imagefile'); % Use "Edit Image" on toolstrip to change.
  Mass Spring : Subsystem  AncestorBlock=Lib/Mass Spring  VariantControl=11ms  mask{m1=2, k1=600, d1=1, s_f=.35, id1=-0.350, zero_forces=off, zerodis=on, force_type=Harmonic, Force=4, Har_Force=2, freq=sqrt(400/1.5)}
      mask prompts: m1 "Mass1 (kg)"; k1 "K1 Spring Constant (N/m)"; d1 "Spring Damping (kg/s)"; s_f "Surface Friction (N/(m/s))"; id1 "M1 Initial Displacement (cm)"; zero_forces "Zero Forces"; zerodis "Zero Initial Displacement"; force_type "Force Response Type"; Force "Magnitude(N)"; Har_Force "Magnitude(N)"; freq "Frequency(rad/s)"
      mask init:
      | switch force_type
      |     case 1
      |         Har_Force = 0;
      |         freq = 0;
      |     case 2
      |         Force = 0;
      | end
      | if zero_forces == 1
      |     Har_Force = 0;
      |     Force = 0;
      |     freq = 0;
      | end
      | 
      | if zerodis == 1
      |     id1 = 0;
      | end
      mask Callback zero_forces:
      | % Enable and disable parameters
      | 
      | % Get the value of the Enable Bias checkbox
      | % unchecked = 'off'
      | % checked = 'on'
      | enab = get_param(gcb,'zero_forces');
      | 
      | % Set the 'MaskEnables' property for each parameters
      | if strcmp(enab,'on')
      |     set_param(gcb,'MaskVisibilities',{'on','on','on','on','on','on','off','off','off','off','off'});
      | else
      |     set_param(gcb,'MaskVisibilities',{'on','on','on','on','on','on','on','on','on','on','on'});
      | end
      | 
      | % Note that the value of the bias is not handled here.
      | % See the Initialization tab
      mask Callback zerodis:
      | % Enable and disable parameters
      | 
      | % Get the value of the Enable Bias checkbox
      | % unchecked = 'off'
      | % checked = 'on'
      | enab = get_param(gcb,'zerodis');
      | 
      | % Set the 'MaskEnables' property for each parameters
      | if strcmp(enab,'on')
      |     set_param(gcb,'MaskEnables',{'on','on','on','on','off','on','on','on','on','on','on'});
      | else
      |     set_param(gcb,'MaskEnables',{'on','on','on','on','on','on','on','on','on','on','on'});
      | end
      | 
      | % Note that the value of the bias is not handled here.
      | % See the Initialization tab
      mask TypeOptions force_type: Step | Harmonic
      mask DialogControl Control4 Prompt: Update Model
      mask DialogControl Control4 Callback: set_param(bdroot,'SimulationCommand','update')
      mask DialogControl Control2 Prompt: Run Simulation
      mask DialogControl Control2 Callback: set_param(bdroot,'SimulationCommand','start')
      mask DialogControl Control3 Prompt: STOP Simulation
      mask DialogControl Control3 Callback: set_param(bdroot,'SimulationCommand','stop')
      mask DialogControl Control7 Prompt: Open Scope Plot
      mask DialogControl Control7 Callback: open(Simulink.BlockPath({'Mass_Springs_Systems/Mass Spring Damper Systems/Mass Spring/Position'}))
      mask DialogControl Container6 Prompt: Variables
      mask DialogControl Container8 Prompt: Free Response
      mask DialogControl Container11 Prompt: Free Response
      mask DialogControl Control10 Prompt: "Check Box below for Only Free Response"
      mask DialogControl Container19 Prompt: Forced Response
      mask DialogControl Container10 Prompt: Forced Response
      mask DialogControl Control9 Prompt: Uncheck "Zero Forces" in Free Response Tab to add Forced Response
      mask DialogControl Container13 Prompt: Step Response
      mask DialogControl Container16 Prompt: Harmonic Response
      mask Display: image('$imagefile'); % Use "Edit Image" on toolstrip to change.
  Spring Mass Spring : Subsystem  AncestorBlock=Lib/Spring Mass Spring  VariantControl=12ms  mask{m1=3, k1=200, k2=600, d=1, s_f=0, id1=1, zero_forces=on, zerodis=off, force_type=Harmonic, Force=3, Har_Force=3, freq=1}
      mask prompts: m1 "Mass1 (kg)"; k1 "K1 Spring Constant (N/m)"; k2 "K2 Spring Constant (N/m)"; d "Spring Damping (kg/s)"; s_f "Surface Friction (N/(m/s))"; id1 "M1 Initial Displacement (cm)"; zero_forces "Zero Forces"; zerodis "Zero Initial Displacement"; force_type "Force Response Type"; Force "Magnitude(N)"; Har_Force "Magnitude(N)"; freq "Frequency(rad/s)"
      mask init:
      | switch force_type
      |     case 1
      |         Har_Force = 0;
      |         freq = 0;
      |     case 2
      |         Force = 0;
      | end
      | if zero_forces == 1
      |     Har_Force = 0;
      |     Force = 0;
      |     freq = 0;
      | end
      | 
      | if zerodis == 1
      |     id1=0;
      | end
      mask Callback zero_forces:
      | % Enable and disable parameters
      | 
      | % Get the value of the Enable Bias checkbox
      | % unchecked = 'off'
      | % checked = 'on'
      | enab = get_param(gcb,'zero_forces');
      | 
      | % Set the 'MaskEnables' property for each parameters
      | if strcmp(enab,'on')
      |     set_param(gcb,'MaskVisibilities',{'on','on','on','on','on','on','on','off','off','off','off','off'});
      | else
      |     set_param(gcb,'MaskVisibilities',{'on','on','on','on','on','on','on','on','on','on','on','on'});
      | end
      | 
      | % Note that the value of the bias is not handled here.
      | % See the Initialization tab
      mask Callback zerodis:
      | % Enable and disable parameters
      | 
      | % Get the value of the Enable Bias checkbox
      | % unchecked = 'off'
      | % checked = 'on'
      | enab = get_param(gcb,'zerodis');
      | 
      | % Set the 'MaskEnables' property for each parameters
      | if strcmp(enab,'on')
      |     set_param(gcb,'MaskEnables',{'on','on','on','on','on','off','on','on','on','on','on','on'});
      | else
      |     set_param(gcb,'MaskEnables',{'on','on','on','on','on','on','on','on','on','on','on','on'});
      | end
      | 
      | % Note that the value of the bias is not handled here.
      | % See the Initialization tab
      mask TypeOptions force_type: Step | Harmonic
      mask DialogControl Control4 Prompt: Update Model
      mask DialogControl Control4 Callback: set_param(bdroot,'SimulationCommand','update')
      mask DialogControl Control2 Prompt: Run Simulation
      mask DialogControl Control2 Callback: set_param(bdroot,'SimulationCommand','start')
      mask DialogControl Control3 Prompt: STOP Simulation
      mask DialogControl Control3 Callback: set_param(bdroot,'SimulationCommand','stop')
      mask DialogControl Control7 Prompt: Open Scope Plot
      mask DialogControl Control7 Callback: open(Simulink.BlockPath({'Mass_Springs_Systems/Mass Spring Damper Systems/Spring Mass Spring/Position'}))
      mask DialogControl Container6 Prompt: Variables
      mask DialogControl Container8 Prompt: Free Response
      mask DialogControl Container11 Prompt: Free Response
      mask DialogControl Control10 Prompt: "Check Box below for Only Free Response"
      mask DialogControl Container19 Prompt: Forced Response
      mask DialogControl Container10 Prompt: Forced Response
      mask DialogControl Control9 Prompt: Uncheck "Zero Forces" in Free Response Tab to add Forced Response
      mask DialogControl Container13 Prompt: Step Response
      mask DialogControl Container16 Prompt: Harmonic Response
      mask Display: image('$imagefile'); % Use "Edit Image" on toolstrip to change.
  Vibrational Machine : Subsystem  Variant=on  VariantControlMode=label  VariantControl=VM  LabelModeActiveChoice=free  mask{togglekc=Input k and c values, rho=100, stiffness=20, flexl=10, M=4000, F=1000000, k2=5000000, c2=10000, v=20, togglem1=Off, m1=500, l1=0.90, togglem2=Off, m2=500, l2=0.90, togglem3=Off, m3=500, l3=0.90, togglem4=Off, m4=500, l4=0.90}
      mask prompts: rho "Density (kg/m^3)"; stiffness "Young's Modulus (GPa)"; flexl "Length (m)"; M "Machine Body Mass (kg)"; F "Force Impulse (N) * 0.2s"; k2 "Calculated system spring stiffness k (N/m)"; c2 "Calculated system spring damping c (N/(m/s))"; v "Angular Velocity (rad/s)"; togglem1 "Mass 1"; m1 "Mass (kg)"; l1 "Distance (m)"; togglem2 "Mass 2"; m2 "Mass (kg)"; l2 "Distance (m)"; togglem3 "Mass 3"; m3 "Mass (kg)"; l3 "Distance (m)"; togglem4 "Mass 4"; m4 "Mass (kg)"; l4 "Distance (m)"
      mask init:
      | switch l1
      |     case 1
      |         l1 = 0.25;
      |     case 2
      |         l1 = 0.5;
      |     case 3
      |         l1 = 0.75;
      |     case 4
      |         l1 = 0.90;
      | end
      | 
      | switch l2
      |     case 1
      |         l2 = 0.25;
      |     case 2
      |         l2 = 0.5;
      |     case 3
      |         l2 = 0.75;
      |     case 4
      |         l2 = 0.90;
      | end
      | 
      | switch l3
      |     case 1
      |         l3 = 0.25;
      |     case 2
      |         l3 = 0.5;
      |     case 3
      |         l3 = 0.75;
      |     case 4
      |         l3 = 0.90;
      | end
      | 
      | switch l4
      |     case 1
      |         l4 = 0.25;
      |     case 2
      |         l4 = 0.5;
      |     case 3
      |         l4 = 0.75;
      |     case 4
      |         l4 = 0.90;
      | end
      | 
      | switch togglekc
      |     case 1
      |     set_param([bdroot '/Mass Spring Damper Systems/Vibrational Machine/Free Vibration/SpringCalc'],'Commented','on');
      |     set_param([bdroot '/Mass Spring Damper Systems/Vibrational Machine/Forced Vibration/SpringCalc'],'Commented','on');
      |     set_param([bdroot '/Mass Spring Damper Systems/Vibrational Machine/Free Vibration/SpringGuess'],'Commented','off');
      |     set_param([bdroot '/Mass Spring Damper Systems/Vibrational Machine/Forced Vibration/SpringGuess'],'Commented','off');
      |     case 2
      |     set_param([bdroot '/Mass Spring Damper Systems/Vibrational Machine/Free Vibration/SpringCalc'],'Commented','off');
      |     set_param([bdroot '/Mass Spring Damper Systems/Vibrational Machine/Forced Vibration/SpringCalc'],'Commented','off');
      |     set_param([bdroot '/Mass Spring Damper Systems/Vibrational Machine/Free Vibration/SpringGuess'],'Commented','on');
      |     set_param([bdroot '/Mass Spring Damper Systems/Vibrational Machine/Forced Vibration/SpringGuess'],'Commented','on');
      | end
      | 
      | switch togglem1
      |     case 1
      |         set_param([bdroot '/Mass Spring Damper Systems/Vibrational Machine/Forced Vibration/Cylindrical Solid2'],'Commented','on');
      |         set_param([bdroot '/Mass Spring Damper Systems/Vibrational Machine/Forced Vibration/Trans1'],'Commented','on');
      |     case 2
      |         set_param([bdroot '/Mass Spring Damper Systems/Vibrational Machine/Forced Vibration/Cylindrical Solid2'],'Commented','off');
      |         set_param([bdroot '/Mass Spring Damper Systems/Vibrational Machine/Forced Vibration/Trans1'],'Commented','off');
      | end
      | 
      | switch togglem2
      |     case 1
      |         set_param([bdroot '/Mass Spring Damper Systems/Vibrational Machine/Forced Vibration/Cylindrical Solid3'],'Commented','on');
      |         set_param([bdroot '/Mass Spring Damper Systems/Vibrational Machine/Forced Vibration/Trans2'],'Commented','on');
      |     case 2
      |         set_param([bdroot '/Mass Spring Damper Systems/Vibrational Machine/Forced Vibration/Cylindrical Solid3'],'Commented','off');
      |         set_param([bdroot '/Mass Spring Damper Systems/Vibrational Machine/Forced Vibration/Trans2'],'Commented','off');
      | end
      | 
      | switch togglem3
      |     case 1
      |         set_param([bdroot '/Mass Spring Damper Systems/Vibrational Machine/Forced Vibration/Cylindrical Solid4'],'Commented','on');
      |         set_param([bdroot '/Mass Spring Damper Systems/Vibrational Machine/Forced Vibration/Trans3'],'Commented','on');
      |     case 2
      |         set_param([bdroot '/Mass Spring Damper Systems/Vibrational Machine/Forced Vibration/Cylindrical Solid4'],'Commented','off');
      |         set_param([bdroot '/Mass Spring Damper Systems/Vibrational Machine/Forced Vibration/Trans3'],'Commented','off');
      | end
      | 
      | switch togglem4
      |     case 1
      |         set_param([bdroot '/Mass Spring Damper Systems/Vibrational Machine/Forced Vibration/Cylindrical Solid5'],'Commented','on');
      |         set_param([bdroot '/Mass Spring Damper Systems/Vibrational Machine/Forced Vibration/Trans4'],'Commented','on');
      |     case 2
      |         set_param([bdroot '/Mass Spring Damper Systems/Vibrational Machine/Forced Vibration/Cylindrical Solid5'],'Commented','off');
      |         set_param([bdroot '/Mass Spring Damper Systems/Vibrational Machine/Forced Vibration/Trans4'],'Commented','off');
      | end
      | 
      | if(togglem1 == 1)
      |     m1 = 0;
      | end
      | 
      | if(togglem2 == 1)
      |     m2 = 0;
      | end
      | 
      | if(togglem3 == 1)
      |     m3 = 0;
      | end
      | 
      | if(togglem4 == 1)
      |     m4 = 0;
      | end
      | 
      | rA = linspace(-pi/2, pi/2, 10)';
      | rB = linspace(pi/2, 3*pi/2, 10)';
      | rC = linspace(3*pi/2, -pi/2, 20)';
      | 
      | r1l = l1;
      | r1w = .2;
      | r1d = .1;
      | r1csRight = [r1l/2 + r1w/2*cos(rA) r1w/2*sin(rA)];
      | r1csLeft = [-r1l/2 + r1w/2*cos(rB) r1w/2*sin(rB)];
      | r1csLeftHole = [-r1l/2 + r1d/2*cos(rC) r1d/2*sin(rC)];
      | r1csRightHole = [r1l/2 + r1d/2*cos(rC) r1d/2*sin(rC)];
      | r1csConnLine = [-r1l/2 -r1w/2; +r1l/2 -r1w/2];
      | r1cs = [r1csRight; r1csLeft; r1csLeftHole; r1csConnLine; r1csRightHole];
      | 
      | %Flexible Beam Properties
      | segl = (flexl-2)/2;
      | width = 1;
      | height = 0.25;
      | bmass = width * height * flexl * rho;
      | E = stiffness*10^9;
      | 
      | %Input forced for equivalent model forced vibration
      | Fcx = (m2*l2-m4*l4)*(v^2);
      | Fcy = (m1*l1-m3*l3)*(v^2);
      | 
      | Meq = M + m1 + m2 + m3 + m4 + 2 + bmass;
      | 
      | %% Run script that reads data file to refine data
      | %% Use output of script to make vibration and damping constant calculations.
      | %% Uncomment this, and enable visibility of toggle button in mask to allow calculations
      | %{ 
      | run('vibtest2.m')
      | 
      | sigma = log(x1/x2);
      | zeta = sigma / (sqrt(4*pi^2 + sigma^2));
      | omegad = 2*pi*(1 / (t2 - t1));
      | omegan = omegad / sqrt(1 - zeta^2);
      | c = 2 * Meq * zeta * omegan;
      | k = omegan^2 * Meq;
      | %}
      | 
      | %% Alternative spring constant calculations
      | %{
      | k3 = (E*(0.25^2))/10;
      | 
      | I = (0.25^4)/12;
      | 
      | k1 = (48*E*I)/(10^3);
      | %}
      | 
      | if(togglekc == 2)
      |     fprintf('Mass Equivalent = %1.3f kg \n Analyzed Spring constant = %1.3f N/m \n Analyzed Damping constant = %1.3f N/(m/s) \n',Meq,k,c);
      | elseif(strcmp(get_param([bdroot '/Mass Spring Damper Systems/Vibrational Machine'],'OverrideUsingVariant'),'free1') == 1)
      |     fprintf('Mass Equivalent = %1.3f kg \n',Meq);
      | else
      |     fprintf('Mass Equivalent = %1.3f kg \n Input Spring constant = %1.3f N/m \n Input Damping constant = %1.3f N/(m/s) \n',Meq,k2,c2);
      | end
      mask TypeOptions togglekc: Input k and c values | Analyze Vibrations
      mask TypeOptions togglem1: Off | On
      mask TypeOptions l1: 0.25 | 0.50 | 0.75 | 0.90
      mask TypeOptions togglem2: Off | On
      mask TypeOptions l2: 0.25 | 0.50 | 0.75 | 0.90
      mask TypeOptions togglem3: Off | On
      mask TypeOptions l3: 0.25 | 0.50 | 0.75 | 0.90
      mask TypeOptions togglem4: Off | On
      mask TypeOptions l4: 0.25 | 0.50 | 0.75 | 0.90
      mask DialogControl Container7 Prompt: Flexible Beam Properties
      mask DialogControl Control11 Prompt: (Keep Low)
      mask DialogControl Container8 Prompt: Machine Properties
      mask DialogControl Control16 Prompt: Check forced vibration tab to see what additional mass is added to the system (Shaft and Disk each have mass of 1 kg).
      mask DialogControl Container5 Prompt: Free Vibration
      mask DialogControl Control2 Prompt: Run Free Vibration
      mask DialogControl Control2 Callback:
      | set_param([bdroot '/Mass Spring Damper Systems/Vibrational Machine'],'OverrideUsingVariant','free1');
      | set_param(bdroot,'SimulationCommand','start');
      mask DialogControl Control9 Prompt: Open Free Vibration Scope
      mask DialogControl Control9 Callback: open_system([bdroot '/Mass Spring Damper Systems/Vibrational Machine/Free Vibration 1/Scope']);
      mask DialogControl Container9 Prompt: Equivalent Model and Characterization
      mask DialogControl Control2_copy Prompt: Run Equivalent Model
      mask DialogControl Control2_copy Callback:
      | set_param([bdroot '/Mass Spring Damper Systems/Vibrational Machine'],'OverrideUsingVariant','free');
      | set_param(bdroot,'SimulationCommand','start');
      mask DialogControl Control9_copy Prompt: Open Equivalent Model Scope
      mask DialogControl Control9_copy Callback: open_system([bdroot '/Mass Spring Damper Systems/Vibrational Machine/Free Vibration/Scope']);
      mask DialogControl Container6 Prompt: Forced Vibration
      mask DialogControl Control3 Prompt: Run Forced Vibration
      mask DialogControl Control3 Callback:
      | set_param([bdroot '/Mass Spring Damper Systems/Vibrational Machine'],'OverrideUsingVariant','force');
      | set_param(bdroot,'SimulationCommand','start');
      mask DialogControl Control10 Prompt: Open Forced Vibration Scope
      mask DialogControl Control10 Callback: open_system([bdroot '/Mass Spring Damper Systems/Vibrational Machine/Forced Vibration/Scope']);
      mask Display: image('$imagefile'); % Use "Edit Image" on toolstrip to change.
